simulink model "Task3"  (R2019b)
settings: Solver=VariableStepAuto  StartTime=0.0  StopTime=20  RelTol=1e-3  EnableMultiTasking=on
settings Model: Creator=zlg12  LastModifiedBy=梁鹏宇
settings DataIOCC: ReturnWorkspaceOutputs=off
settings OptimizationCC: LifeSpan=inf
settings DebuggingCC: SFUnexpectedBacktrackingDiag=warning  SFNoUnconditionalDefaultTransitionDiag=warning  ArithmeticOperatorsInVariantConditions=warning
settings SFSimCC: SimUseLocalCustomCode=off  CustomCodeUndefinedFunction=UseInterfaceOnly
settings RTWCC: RTWUseLocalCustomCode=off
settings CodeAppCC: StateflowObjectComments=on
settings GRTTargetCC: TargetLangStandard=C89/C90 (ANSI)  GeneratePreprocessorConditionals=Disable all
settings ConfigComp: CovMetricSettings=dw  CovHtmlReporting=on  CovSaveCumulativeToWorkspaceVar=on  CovSaveSingleToWorkspaceVar=on  CovExternalEMLEnable=off

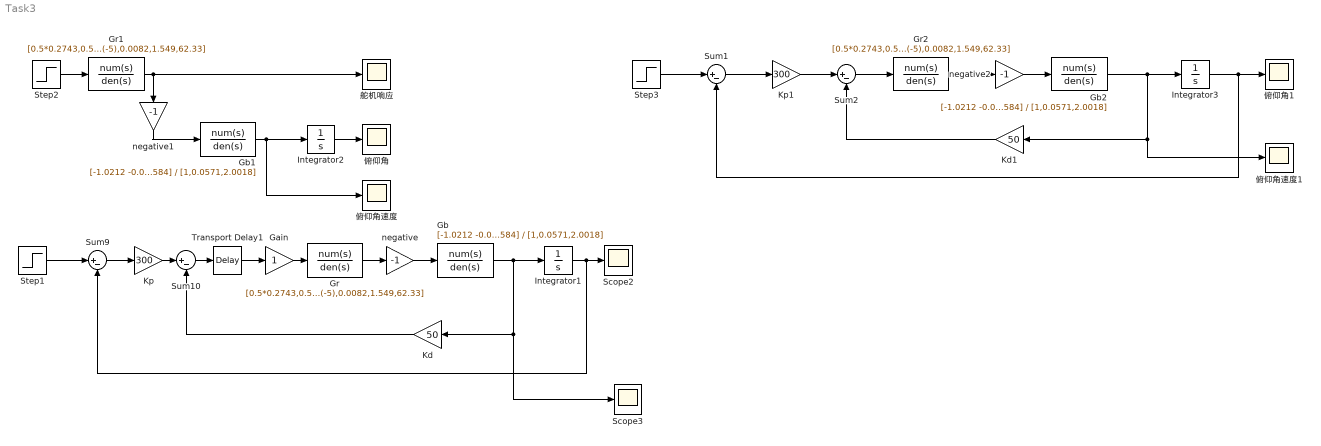
== system Task3 ==
  Gain : Gain
  Gb : TransferFcn  Numerator=[-1.0212 -0.0584]  Denominator=[1,0.0571,2.0018]
  Gb1 : TransferFcn  Numerator=[-1.0212 -0.0584]  Denominator=[1,0.0571,2.0018]
  Gb2 : TransferFcn  Numerator=[-1.0212 -0.0584]  Denominator=[1,0.0571,2.0018]
  Gr : TransferFcn  Numerator=[0.5*0.2743,0.5*124.7]  Denominator=[1.32*10^(-5),0.0082,1.549,62.33]
  Gr1 : TransferFcn  Numerator=[0.5*0.2743,0.5*124.7]  Denominator=[1.32*10^(-5),0.0082,1.549,62.33]
  Gr2 : TransferFcn  Numerator=[0.5*0.2743,0.5*124.7]  Denominator=[1.32*10^(-5),0.0082,1.549,62.33]
  Integrator1 : Integrator
  Integrator2 : Integrator
  Integrator3 : Integrator
  Kd : Gain  Gain=50
  Kd1 : Gain  Gain=50
  Kp : Gain  Gain=300
  Kp1 : Gain  Gain=300
  Scope2 : Scope
  "Scope3 " : Scope
  Step1 : Step  Time=0  SampleTime=0
  Step2 : Step  Time=0  SampleTime=0
  Step3 : Step  Time=0  SampleTime=0
  Sum{1..2,9..10} (4 alike) : Sum  Inputs=|+-
  Transport Delay1 : TransportDelay  DelayTime=0
  negative : Gain  Gain=-1
  negative1 : Gain  Gain=-1
  negative2 : Gain  Gain=-1
  俯仰角 : Scope
  俯仰角1 : Scope
  俯仰角速度 : Scope
  俯仰角速度1 : Scope
  舵机响应 : Scope
  wires:
  Step1/1 -> Sum9/1
  Sum9/1 -> Kp/1
  Kd/1 -> Sum10/2
  Kp/1 -> Sum10/1
  negative/1 -> Gb/1
  Integrator1/1 -> Sum9/2, Scope2/1
  Gb/1 -> Integrator1/1, "Scope3 "/1, Kd/1
  Gr/1 -> negative/1
  Step2/1 -> Gr1/1
  Gr1/1 -> negative1/1, 舵机响应/1
  Integrator2/1 -> 俯仰角/1
  Gb1/1 -> 俯仰角速度/1, Integrator2/1
  Sum10/1 -> Transport Delay1/1
  Transport Delay1/1 -> Gain/1
  Gain/1 -> Gr/1
  negative1/1 -> Gb1/1
  Step3/1 -> Sum1/1
  Sum1/1 -> Kp1/1
  Kp1/1 -> Sum2/1
  Sum2/1 -> Gr2/1
  Gr2/1 -> negative2/1
  negative2/1 -> Gb2/1
  Gb2/1 -> 俯仰角速度1/1, Kd1/1, Integrator3/1
  Kd1/1 -> Sum2/2
  Integrator3/1 -> Sum1/2, 俯仰角1/1
